simulink model "chap1_27"  (Simulink 6.3)
settings: Solver=ode45  StartTime=0.0  StopTime=10  RelTol=1e-3
undefined symbols (not defined in the file or in its folder): chap1_27f
settings Model: Creator=hp  LastModifiedBy=Administrator  ExtModeTrigMode=oneshot  ExtModeArmWhenConnect=off
settings DataIOCC: LimitDataPoints=off
settings OptimizationCC: BlockReduction=off  BooleanDataType=off
settings DebuggingCC: SolverPrmCheckMsg=none
settings HardwareCC: TargetUnknown=on

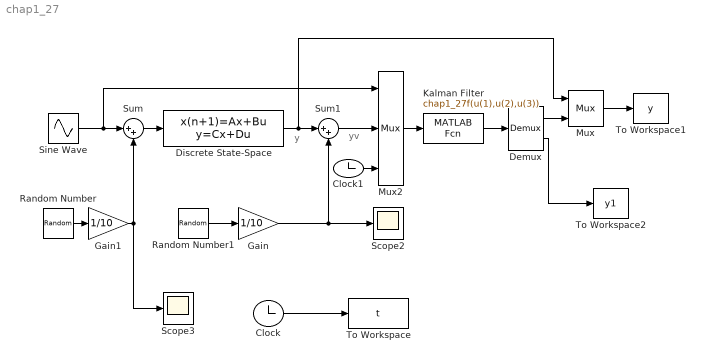
== system chap1_27 ==
  note: y
  note: yv
  Clock : Clock
      settings: Decimation=10
  Clock1 : Clock
  Demux : Demux  Outputs=2
  Discrete State-Space : DiscreteStateSpace  A=[1.0000 0.0010;0 0.9753]  B=[0.0001;0.1314]  C=[1 0]  D=0  SampleTime=0.001
  Gain : Gain  Gain=1/10  SaturateOnIntegerOverflow=on
  Gain1 : Gain  Gain=1/10  SaturateOnIntegerOverflow=on
  Kalman Filter : MATLABFcn  MATLABFcn=chap1_27f(u(1),u(2),u(3))  OutputDimensions=2
  Mux : Mux  Inputs=2
  Mux2 : Mux  Inputs=3
  Random Number : RandomNumber  SampleTime=0.001
  Random Number1 : RandomNumber  SampleTime=0.001
  Scope2 : Scope
      settings: TimeRange=1  YMin=-3  YMax=3.5
  Scope3 : Scope
      settings: TimeRange=1  YMin=-3  YMax=2
  Sine Wave : Sin  Frequency=1*pi  SampleTime=0.001
  Sum : Sum  Inputs=|++  SaturateOnIntegerOverflow=on  InputSameDT=on
  Sum1 : Sum  Inputs=|++  SaturateOnIntegerOverflow=on  InputSameDT=on
  To Workspace : ToWorkspace  VariableName=t  SampleTime=-1  SaveFormat=Array
  To Workspace1 : ToWorkspace  VariableName=y  SampleTime=-1  SaveFormat=Array
  To Workspace2 : ToWorkspace  VariableName=y1  SampleTime=-1  SaveFormat=Array
  wires:
  Mux2/1 -> Kalman Filter/1
  Clock1/1 -> Mux2/3
  Sine Wave/1 -> Mux2/1, Sum/1
  Sum/1 -> Discrete State-Space/1
  Sum1/1 -> Mux2/2
  Discrete State-Space/1 -> Sum1/1, Mux/1
  Random Number/1 -> Gain1/1
  Kalman Filter/1 -> Demux/1
  Gain1/1 -> Sum/2, Scope3/1
  Random Number1/1 -> Gain/1
  Gain/1 -> Sum1/2, Scope2/1
  Demux/2 -> To Workspace2/1
  Demux/1 -> Mux/2
  Mux/1 -> To Workspace1/1
  Clock/1 -> To Workspace/1
